simulink model "AutonomousTest1"  (R2021b)
settings: Solver=FixedStepAuto  StartTime=0.0  StopTime=inf  RelTol=1e-3
libraries: vexarmcortexlib x26, simulink x8, vexcommonlib x1
settings Model: SimulationMode=external  NumberOfSteps=6  Creator=arago  LastModifiedBy=arago
settings DataIOCC: LimitDataPoints=on  SignalLoggingSaveFormat=ModelDataLogs  ReturnWorkspaceOutputs=off
settings OptimizationCC: ExpressionDepthLimit=2147483647  LifeSpan=Inf  MaxStackSize=64  EfficientTunableParamExpr=on
settings DebuggingCC: UnderspecifiedInitializationDetection=Classic  MergeDetectMultiDrivingBlocksExec=none  InheritedTsInSrcMsg=none  FcnCallInpInsideContextMsg=warning  UnconnectedInputMsg=none  UnconnectedOutputMsg=none  StateNameClashWarn=warning  SFUnexpectedBacktrackingDiag=warning  SFNoUnconditionalDefaultTransitionDiag=warning  SFExecutionAtInitializationDiag=none  SFMachineParentedDataDiag=warning  ArithmeticOperatorsInVariantConditions=warning
settings HardwareCC: ProdBitPerPointer=32  ProdBitPerSizeT=32  ProdBitPerPtrDiffT=32  ProdLargestAtomicInteger=Long  ProdLargestAtomicFloat=Double  ProdIntDivRoundTo=Undefined  ProdWordSize=32  ProdHWDeviceType=ARM Compatible->ARM Cortex
settings ModelReferenceCC: PropagateSignalLabelsOutOfModel=off
settings SFSimCC: MATLABDynamicMemAlloc=off  CustomCodeUndefinedFunction=UseInterfaceOnly
settings RTWCC: Description=Embedded Coder  SystemTargetFile=ert.tlc  HardwareBoard=ARM Cortex-based VEX Microcontroller  TemplateMakefile=ert_default_tmf  Toolchain=GNU Tools for VEX ARM Cortex
settings CodeAppCC: IgnoreCustomStorageClasses=off  CustomSymbolStrType=$N$R$M  StateflowObjectComments=on  InternalIdentifier=Classic
settings ERTTargetCC: CodeReplacementLibrary=GCC ARM Cortex-M3  MultiwordLength=2048  ConvertIfToSwitch=off  SuppressUnreachableDefaultCases=off

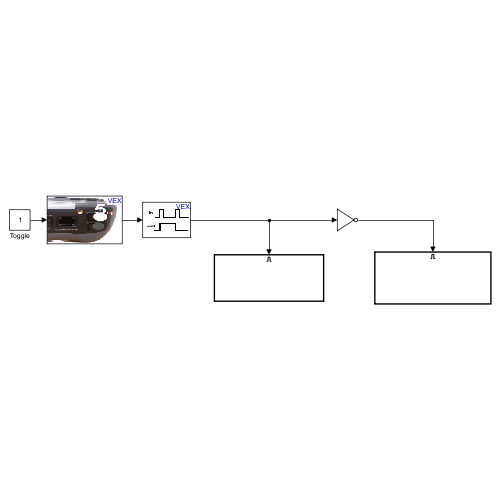
[thumbnail: Simulink's stored preview of the top-level diagram]
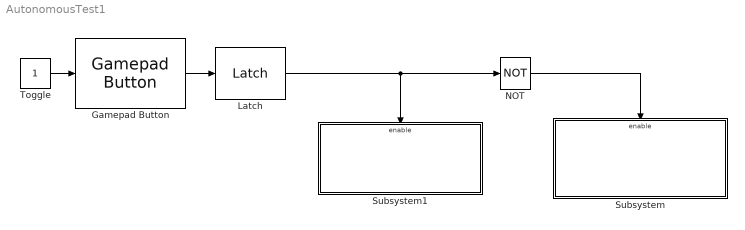
== system AutonomousTest1 ==
  Gamepad Button : vexarmcortexlib/Gamepad/Gamepad Button  joystick=1  chan=5  button56=Up  button78=Left  SimulationIn=on  SampleTime=0.02
      settings: SourceProductBaseCode=EC_VEX_MICRO
  Latch : vexcommonlib/Latch  output0=off  BlockPlatform=vexarmcortex
      settings: SourceProductBaseCode=EC_VEX_MICRO,VEXV5
  NOT : Logic  Operator=NOT  IconShape=distinctive  AllPortsSameDT=off  OutDataTypeStr=boolean
  Subsystem : Subsystem
  Subsystem1 : Subsystem
  Toggle : Constant
      settings: OpenFcn=|
      | if strcmp('0',get_param(gcb, 'Value'))                        set_param(gcb, 'Value', '1');
      | else
      |             set_param(gcb, 'Value', '0');
      | end
  wires:
  NOT/1 -> Subsystem/Enable
  Latch/1 -> Subsystem1/Enable, NOT/1
  Gamepad Button/1 -> Latch/1
  Toggle/1 -> Gamepad Button/1

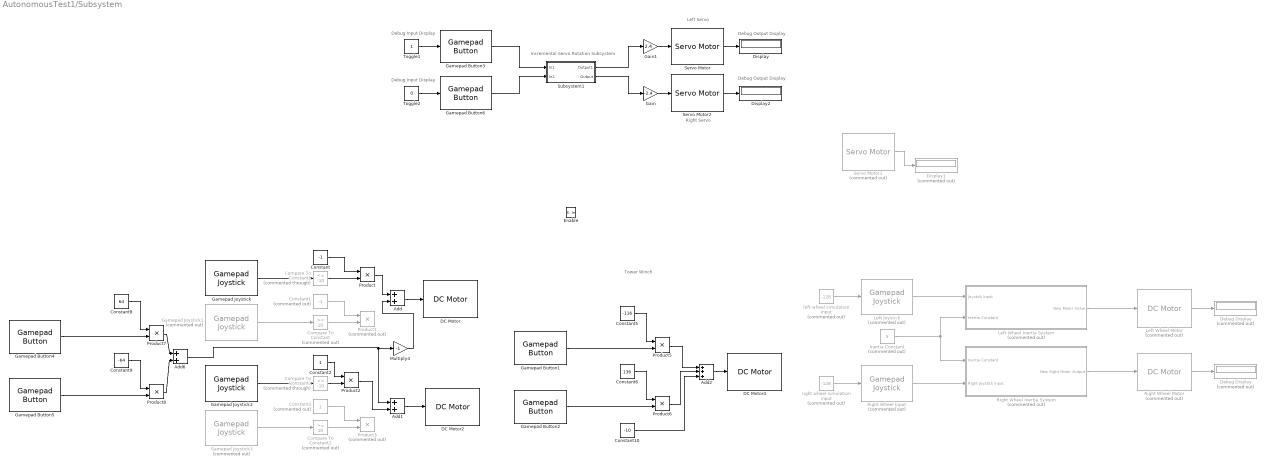
== system AutonomousTest1/Subsystem ==
  note: Incremental Servo Rotation Subsystem
  note: Left Servo
  note: Tower Winch
  note: Right Servo
  note: Debug Output Display
  note: Debug Output Display
  note: Debug Input Display
  note: Debug Input Display
  Enable : EnablePort
  " Debug Display" : Display  Commented=on
  Add : Sum
  Add1 : Sum
  Add2 : Sum  Inputs=+++
  Add6 : Sum
  Compare To Constant : simulink/Logic and Bit Operations/Compare To Constant  Commented=on  relop=>=  const=10  OutDataTypeStr=uint8
  Compare To Constant1 : simulink/Logic and Bit Operations/Compare To Constant  Commented=through  relop=<=  const=-10  OutDataTypeStr=uint8
  Compare To Constant2 : simulink/Logic and Bit Operations/Compare To Constant  Commented=on  relop=>=  const=10  OutDataTypeStr=uint8
  Compare To Constant3 : simulink/Logic and Bit Operations/Compare To Constant  Commented=through  relop=<=  const=-10  OutDataTypeStr=uint8
  Constant : Constant  Value=-1
  Constant1 : Constant  Commented=on  Value=-1
  Constant10 : Constant  Value=-10
  Constant2 : Constant
  Constant3 : Constant  Commented=on
  Constant5 : Constant  Value=-116
  Constant6 : Constant  Value=136
  Constant8 : Constant  Value=64
  Constant9 : Constant  Value=-64
  DC Motor : vexarmcortexlib/Actuators/DC Motor  motor=2  scaleFactor=1/13.5  SimulationOut=off
      settings: SourceProductBaseCode=EC_VEX_MICRO
  DC Motor2 : vexarmcortexlib/Actuators/DC Motor  motor=3  scaleFactor=1/13.5  SimulationOut=off
      settings: SourceProductBaseCode=EC_VEX_MICRO
  DC Motor4 : vexarmcortexlib/Actuators/DC Motor  motor=6  scaleFactor=1/13.5  SimulationOut=off
      settings: SourceProductBaseCode=EC_VEX_MICRO
  Debug Display : Display  Commented=on
  Display : Display
  Display1 : Display  Commented=on
  Display2 : Display
  Gain : Gain  Gain=-2.4
  Gain1 : Gain  Gain=2.4
  Gamepad Button1 : vexarmcortexlib/Gamepad/Gamepad Button  joystick=1  chan=8  button56=Up  button78=Up  SimulationIn=off  SampleTime=0.02
      settings: SourceProductBaseCode=EC_VEX_MICRO
  Gamepad Button2 : vexarmcortexlib/Gamepad/Gamepad Button  joystick=1  chan=8  button56=Up  button78=Down  SimulationIn=off  SampleTime=0.02
      settings: SourceProductBaseCode=EC_VEX_MICRO
  Gamepad Button3 : vexarmcortexlib/Gamepad/Gamepad Button  joystick=1  chan=6  button56=Up  button78=Down  SimulationIn=on  SampleTime=0.02
      settings: SourceProductBaseCode=EC_VEX_MICRO
  Gamepad Button4 : vexarmcortexlib/Gamepad/Gamepad Button  joystick=1  chan=7  button56=Up  button78=Up  SimulationIn=off  SampleTime=0.02
      settings: SourceProductBaseCode=EC_VEX_MICRO
  Gamepad Button5 : vexarmcortexlib/Gamepad/Gamepad Button  joystick=1  chan=7  button56=Up  button78=Down  SimulationIn=off  SampleTime=0.02
      settings: SourceProductBaseCode=EC_VEX_MICRO
  Gamepad Button6 : vexarmcortexlib/Gamepad/Gamepad Button  joystick=1  chan=6  button56=Down  button78=Down  SimulationIn=on  SampleTime=0.02
      settings: SourceProductBaseCode=EC_VEX_MICRO
  Gamepad Joystick : vexarmcortexlib/Gamepad/Gamepad Joystick  joystick=1  chan=2  SimulationIn=off  SampleTime=0.02
      settings: SourceProductBaseCode=EC_VEX_MICRO
  Gamepad Joystick1 : vexarmcortexlib/Gamepad/Gamepad Joystick  Commented=on  joystick=1  chan=2  SimulationIn=off  SampleTime=0.02
      settings: SourceProductBaseCode=EC_VEX_MICRO
  Gamepad Joystick2 : vexarmcortexlib/Gamepad/Gamepad Joystick  joystick=1  chan=3  SimulationIn=off  SampleTime=0.02
      settings: SourceProductBaseCode=EC_VEX_MICRO
  Gamepad Joystick3 : vexarmcortexlib/Gamepad/Gamepad Joystick  Commented=on  joystick=1  chan=3  SimulationIn=off  SampleTime=0.02
      settings: SourceProductBaseCode=EC_VEX_MICRO
  Inertia Constant : Constant  Commented=on  Value=5
  Left Joystick : vexarmcortexlib/Gamepad/Gamepad Joystick  Commented=on  joystick=1  chan=3  SimulationIn=on  SampleTime=0.02
      settings: SourceProductBaseCode=EC_VEX_MICRO
  Left Wheel Inertia System : Subsystem  Commented=on
  Left Wheel Motor : vexarmcortexlib/Actuators/DC Motor  Commented=on  motor=2  scaleFactor=1/13.5  SimulationOut=on
      settings: SourceProductBaseCode=EC_VEX_MICRO
  Multiply4 : Gain  Gain=-1
  Product{,2,5..8} (6 alike) : Product
  Product1 : Product  Commented=on
  Product3 : Product  Commented=on
  Right Wheel Inertia System : Subsystem  Commented=on
  Right Wheel Input : vexarmcortexlib/Gamepad/Gamepad Joystick  Commented=on  joystick=1  chan=2  SimulationIn=on  SampleTime=0.02
      settings: SourceProductBaseCode=EC_VEX_MICRO
  Right Wheel Motor : vexarmcortexlib/Actuators/DC Motor  Commented=on  motor=3  scaleFactor=1/13.5  SimulationOut=on
      settings: SourceProductBaseCode=EC_VEX_MICRO
  Servo Motor : vexarmcortexlib/Actuators/Servo Motor  motor=5  scaleFactor=60/127  SimulationOut=on
      settings: SourceProductBaseCode=EC_VEX_MICRO
  Servo Motor1 : vexarmcortexlib/Actuators/Servo Motor  Commented=on  motor=5  scaleFactor=60/127  SimulationOut=on
      settings: SourceProductBaseCode=EC_VEX_MICRO
  Servo Motor2 : vexarmcortexlib/Actuators/Servo Motor  motor=4  scaleFactor=60/127  SimulationOut=on
      settings: SourceProductBaseCode=EC_VEX_MICRO
  Subsystem1 : Subsystem
  Toggle1 : Constant
      settings: OpenFcn=|
      | if strcmp('0',get_param(gcb, 'Value'))                        set_param(gcb, 'Value', '1');
      | else
      |             set_param(gcb, 'Value', '0');
      | end
  Toggle2 : Constant  Value=0
      settings: OpenFcn=|
      | if strcmp('0',get_param(gcb, 'Value'))                        set_param(gcb, 'Value', '1');
      | else
      |             set_param(gcb, 'Value', '0');
      | end
  left wheel simulation input : Constant  Commented=on  Value=-128  SampleTime=0.02
  right wheel simulation input : Constant  Commented=on  Value=-128  SampleTime=0.02
  wires:
  Constant6/1 -> Product6/1
  Constant2/1 -> Product2/1
  Subsystem1/1(Output1) -> Gain1/1
  Constant10/1 -> Add2/3
  Gamepad Joystick1/1 -> Compare To Constant/1
  Product5/1 -> Add2/1
  Constant8/1 -> Product7/1
  Compare To Constant1/1 -> Product/2
  Gamepad Button3/1 -> Subsystem1/1(In1)
  Constant1/1 -> Product1/1
  Right Wheel Motor/1 -> Debug Display/1
  Constant5/1 -> Product5/1
  Servo Motor2/1 -> Display2/1
  Gamepad Joystick/1 -> Compare To Constant1/1
  right wheel simulation input/1 -> Right Wheel Input/1
  Product6/1 -> Add2/2
  left wheel simulation input/1 -> Left Joystick/1
  Servo Motor/1 -> Display/1
  Product2/1 -> Add1/2
  Gamepad Joystick3/1 -> Compare To Constant2/1
  Constant9/1 -> Product8/1
  Gamepad Button2/1 -> Product6/2
  Product/1 -> Add/1
  Compare To Constant/1 -> Product1/2
  Add2/1 -> DC Motor4/1
  Gamepad Button6/1 -> Subsystem1/2(In2)
  Compare To Constant2/1 -> Product3/2
  Left Wheel Motor/1 -> " Debug Display"/1
  Servo Motor1/1 -> Display1/1
  Constant/1 -> Product/1
  Add6/1 -> Multiply4/1, Add1/1
  Gamepad Button1/1 -> Product5/2
  Gamepad Joystick2/1 -> Compare To Constant3/1
  Compare To Constant3/1 -> Product2/2
  Product8/1 -> Add6/2
  Subsystem1/2(Output) -> Gain/1
  Product7/1 -> Add6/1
  Gain/1 -> Servo Motor2/1
  Constant3/1 -> Product3/1
  Inertia Constant/1 -> Right Wheel Inertia System/1(Inertia Constant), Left Wheel Inertia System/2(Inertia Constant)
  Gain1/1 -> Servo Motor/1
  Left Joystick/1 -> Left Wheel Inertia System/1(Joystick Input)
  Gamepad Button4/1 -> Product7/2
  Right Wheel Input/1 -> Right Wheel Inertia System/2(Right Joystick Input)
  Right Wheel Inertia System/1(New Right Motor Output) -> Right Wheel Motor/1
  Toggle2/1 -> Gamepad Button6/1
  Toggle1/1 -> Gamepad Button3/1
  Left Wheel Inertia System/1(New Motor Value) -> Left Wheel Motor/1
  Add1/1 -> DC Motor2/1
  Add/1 -> DC Motor/1
  Multiply4/1 -> Add/2
  Gamepad Button5/1 -> Product8/2

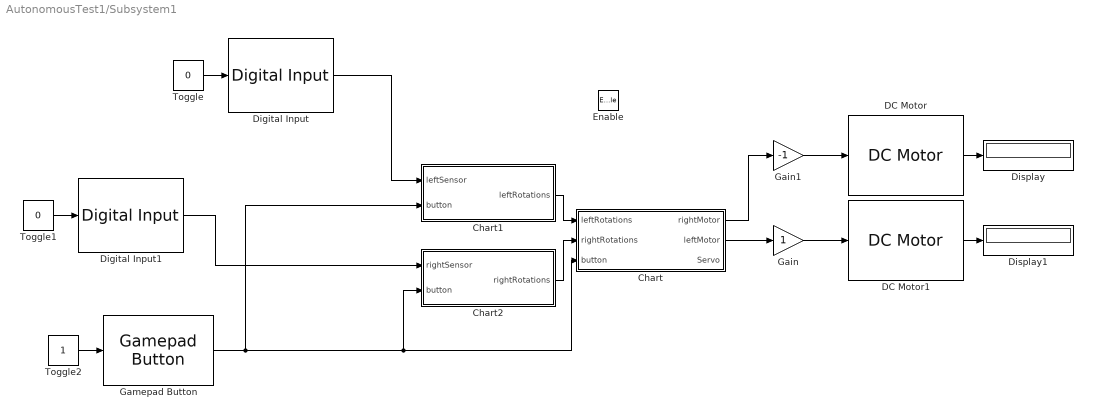
== system AutonomousTest1/Subsystem1 ==
  Enable : EnablePort
  Chart : Stateflow chart  TreatAsAtomicUnit=on
  Chart1 : Stateflow chart  TreatAsAtomicUnit=on
  Chart2 : Stateflow chart  TreatAsAtomicUnit=on
  DC Motor : vexarmcortexlib/Actuators/DC Motor  motor=2  scaleFactor=1/13.5  SimulationOut=on
      settings: SourceProductBaseCode=EC_VEX_MICRO
  DC Motor1 : vexarmcortexlib/Actuators/DC Motor  motor=3  scaleFactor=1/13.5  SimulationOut=on
      settings: SourceProductBaseCode=EC_VEX_MICRO
  Digital Input : vexarmcortexlib/Sensors/Digital Input  inChan=1  SimulationIn=on  SampleTime=.05
      settings: SourceProductBaseCode=EC_VEX_MICRO
  Digital Input1 : vexarmcortexlib/Sensors/Digital Input  inChan=2  SimulationIn=on  SampleTime=.05
      settings: SourceProductBaseCode=EC_VEX_MICRO
  Display : Display
  Display1 : Display
  Gain : Gain
  Gain1 : Gain  Gain=-1
  Gamepad Button : vexarmcortexlib/Gamepad/Gamepad Button  joystick=1  chan=5  button56=Up  button78=Left  SimulationIn=on  SampleTime=0.02
      settings: SourceProductBaseCode=EC_VEX_MICRO
  Toggle : Constant  Value=0
      settings: OpenFcn=|
      | if strcmp('0',get_param(gcb, 'Value'))                        set_param(gcb, 'Value', '1');
      | else
      |             set_param(gcb, 'Value', '0');
      | end
  Toggle1 : Constant  Value=0
      settings: OpenFcn=|
      | if strcmp('0',get_param(gcb, 'Value'))                        set_param(gcb, 'Value', '1');
      | else
      |             set_param(gcb, 'Value', '0');
      | end
  Toggle2 : Constant
      settings: OpenFcn=|
      | if strcmp('0',get_param(gcb, 'Value'))                        set_param(gcb, 'Value', '1');
      | else
      |             set_param(gcb, 'Value', '0');
      | end
  wires:
  Digital Input/1 -> Chart1/1(leftSensor)
  Chart1/1(leftRotations) -> Chart/1(leftRotations)
  Digital Input1/1 -> Chart2/1(rightSensor)
  Chart2/1(rightRotations) -> Chart/2(rightRotations)
  Gamepad Button/1 -> Chart2/2(button), Chart/3(button), Chart1/2(button)
  Toggle1/1 -> Digital Input1/1
  DC Motor/1 -> Display/1
  DC Motor1/1 -> Display1/1
  Chart/2(leftMotor) -> Gain/1
  Gain/1 -> DC Motor1/1
  Gain1/1 -> DC Motor/1
  Chart/1(rightMotor) -> Gain1/1
  Toggle2/1 -> Gamepad Button/1
  Toggle/1 -> Digital Input/1

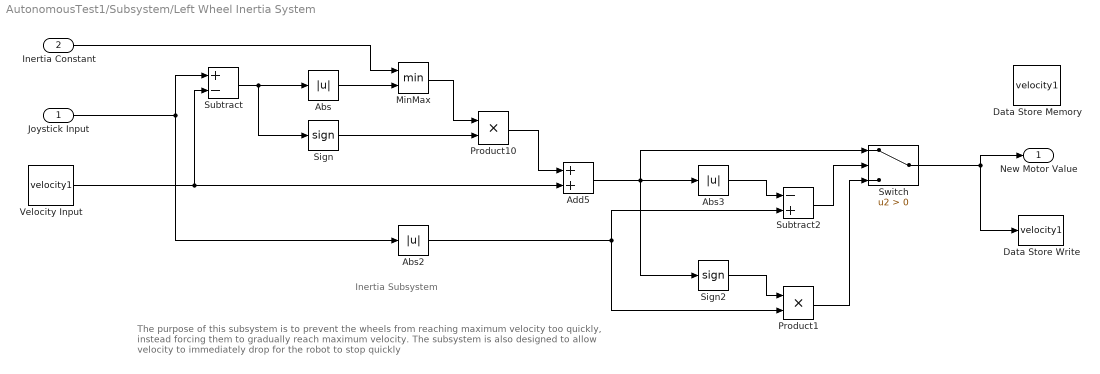
== system AutonomousTest1/Subsystem/Left Wheel Inertia System ==
  note: The purpose of this subsystem is to prevent the wheels from reaching maximum velocity too quickly, instead forcing them to gradually reach maximum velocity. The subsystem is also designed to allow velocity to immediately drop for the robot to stop quickly
  note: Inertia Subsystem
  Joystick Input : Inport
  Inertia Constant : Inport  Port=2
  Abs : Abs
  Abs2 : Abs
  Abs3 : Abs
  Add5 : Sum
  Data Store Memory : DataStoreMemory  DataStoreName=velocity1  ReadBeforeWriteMsg=warning  WriteAfterWriteMsg=warning  WriteAfterReadMsg=warning  ShowAdditionalParam=off
  Data Store Write : DataStoreWrite  DataStoreName=velocity1  SampleTime=0.02  IndexOptions=Index vector (dialog)  Indices=1  OutputSizes=1
  MinMax : MinMax  Inputs=2
  Product1 : Product  RndMeth=Zero
  Product10 : Product  RndMeth=Zero
  Sign : Signum
  Sign2 : Signum
  Subtract : Sum  Inputs=+-
  Subtract2 : Sum  Inputs=-+
  Switch : Switch  Criteria=u2 > Threshold
  Velocity Input : DataStoreRead  DataStoreName=velocity1  SampleTime=0.02  IndexOptions=Index vector (dialog)  Indices=1  OutputSizes=1
  New Motor Value : Outport
  wires:
  Joystick Input/1 -> Subtract/1, Abs2/1
  Subtract/1 -> Sign/1, Abs/1
  Add5/1 -> Sign2/1, Switch/1, Abs3/1
  Abs/1 -> MinMax/2
  Sign/1 -> Product10/2
  Velocity Input/1 -> Subtract/2, Add5/2
  Abs2/1 -> Subtract2/2, Product1/2
  Product10/1 -> Add5/1
  Sign2/1 -> Product1/1
  MinMax/1 -> Product10/1
  Inertia Constant/1 -> MinMax/1
  Switch/1 -> New Motor Value/1, Data Store Write/1
  Subtract2/1 -> Switch/2
  Abs3/1 -> Subtract2/1
  Product1/1 -> Switch/3

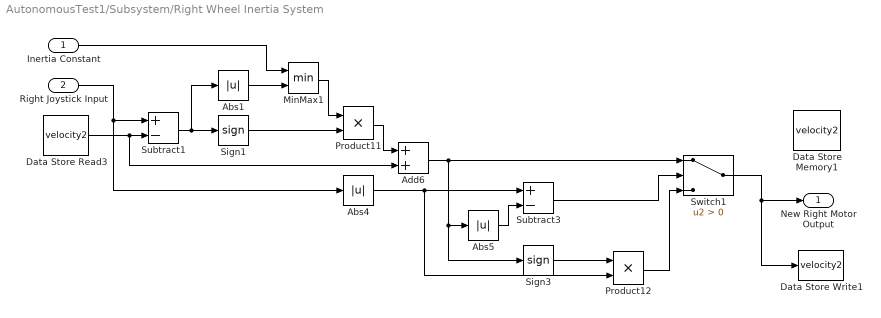
== system AutonomousTest1/Subsystem/Right Wheel Inertia System ==
  Inertia Constant : Inport
  Right Joystick Input : Inport  Port=2
  Abs1 : Abs
  Abs4 : Abs
  Abs5 : Abs
  Add6 : Sum
  Data Store Memory1 : DataStoreMemory  DataStoreName=velocity2  ReadBeforeWriteMsg=warning  WriteAfterWriteMsg=warning  WriteAfterReadMsg=warning  ShowAdditionalParam=off
  Data Store Read3 : DataStoreRead  DataStoreName=velocity2  SampleTime=0.02  IndexOptions=Index vector (dialog)  Indices=1  OutputSizes=1
  Data Store Write1 : DataStoreWrite  DataStoreName=velocity2  SampleTime=0.02  IndexOptions=Index vector (dialog)  Indices=1  OutputSizes=1
  MinMax1 : MinMax  Inputs=2
  Product11 : Product  RndMeth=Zero
  Product12 : Product  RndMeth=Zero
  Sign1 : Signum
  Sign3 : Signum
  Subtract1 : Sum  Inputs=+-
  Subtract3 : Sum  Inputs=+-
  Switch1 : Switch  Criteria=u2 > Threshold
  New Right Motor Output : Outport
  wires:
  MinMax1/1 -> Product11/1
  Abs5/1 -> Subtract3/2
  Product11/1 -> Add6/1
  Abs4/1 -> Product12/2, Subtract3/1
  Abs1/1 -> MinMax1/2
  Subtract3/1 -> Switch1/2
  Subtract1/1 -> Abs1/1, Sign1/1
  Sign1/1 -> Product11/2
  Sign3/1 -> Product12/1
  Data Store Read3/1 -> Subtract1/2, Add6/2
  Add6/1 -> Abs5/1, Sign3/1, Switch1/1
  Right Joystick Input/1 -> Abs4/1, Subtract1/1
  Inertia Constant/1 -> MinMax1/1
  Product12/1 -> Switch1/3
  Switch1/1 -> Data Store Write1/1, New Right Motor Output/1

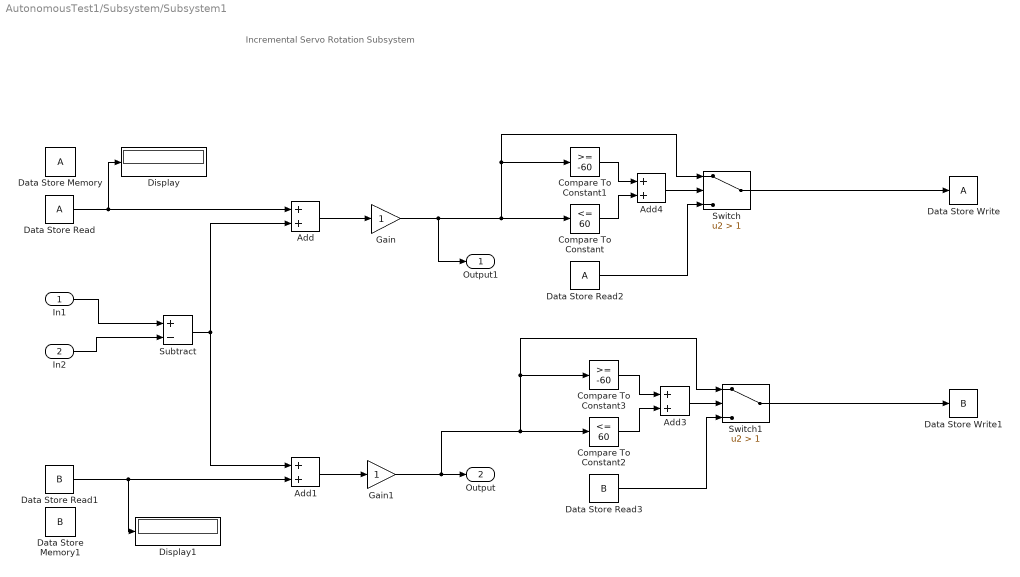
== system AutonomousTest1/Subsystem/Subsystem1 ==
  note: Incremental Servo Rotation Subsystem
  In1 : Inport
  In2 : Inport  Port=2
  Add{,1,3..4} (4 alike) : Sum
  Compare To Constant : simulink/Logic and Bit Operations/Compare To Constant  relop=<=  const=60  OutDataTypeStr=boolean
  Compare To Constant1 : simulink/Logic and Bit Operations/Compare To Constant  relop=>=  const=-60  OutDataTypeStr=boolean
  Compare To Constant2 : simulink/Logic and Bit Operations/Compare To Constant  relop=<=  const=60  OutDataTypeStr=boolean
  Compare To Constant3 : simulink/Logic and Bit Operations/Compare To Constant  relop=>=  const=-60  OutDataTypeStr=boolean
  Data Store Memory : DataStoreMemory  ReadBeforeWriteMsg=warning  WriteAfterWriteMsg=warning  WriteAfterReadMsg=warning  ShowAdditionalParam=off
  Data Store Memory1 : DataStoreMemory  DataStoreName=B  ReadBeforeWriteMsg=warning  WriteAfterWriteMsg=warning  WriteAfterReadMsg=warning  ShowAdditionalParam=off
  Data Store Read : DataStoreRead  IndexOptions=Index vector (dialog)  Indices=1  OutputSizes=1
  Data Store Read1 : DataStoreRead  DataStoreName=B  IndexOptions=Index vector (dialog)  Indices=1  OutputSizes=1
  Data Store Read2 : DataStoreRead  IndexOptions=Index vector (dialog)  Indices=1  OutputSizes=1
  Data Store Read3 : DataStoreRead  DataStoreName=B  IndexOptions=Index vector (dialog)  Indices=1  OutputSizes=1
  Data Store Write : DataStoreWrite  IndexOptions=Index vector (dialog)  Indices=1  OutputSizes=1
  Data Store Write1 : DataStoreWrite  DataStoreName=B  IndexOptions=Index vector (dialog)  Indices=1  OutputSizes=1
  Display : Display
  Display1 : Display
  Gain : Gain
  Gain1 : Gain
  Subtract : Sum  Inputs=+-
  Switch : Switch  Criteria=u2 > Threshold  Threshold=1
  Switch1 : Switch  Criteria=u2 > Threshold  Threshold=1
  Output1 : Outport
  Output : Outport  Port=2
  wires:
  In1/1 -> Subtract/1
  Add/1 -> Gain/1
  Add1/1 -> Gain1/1
  In2/1 -> Subtract/2
  Subtract/1 -> Add1/1, Add/2
  Gain/1 -> Compare To Constant1/1, Switch/1, Compare To Constant/1, Output1/1
  Switch/1 -> Data Store Write/1
  Switch1/1 -> Data Store Write1/1
  Data Store Read/1 -> Display/1, Add/1
  Data Store Read1/1 -> Display1/1, Add1/2
  Compare To Constant1/1 -> Add4/1
  Compare To Constant/1 -> Add4/2
  Add4/1 -> Switch/2
  Data Store Read2/1 -> Switch/3
  Compare To Constant2/1 -> Add3/2
  Data Store Read3/1 -> Switch1/3
  Add3/1 -> Switch1/2
  Compare To Constant3/1 -> Add3/1
  Gain1/1 -> Compare To Constant3/1, Switch1/1, Compare To Constant2/1, Output/1

== stateflow chart AutonomousTest1/Subsystem1/Chart ==
  state CloseClaw
    leftMotor = 0;
    rightMotor= 0;
    Servo = 0;
  state Straight
    leftMotor = 100;
    rightMotor = 100;
  state DriveForward
    leftMotor = 100;
    rightMotor = 100;
  state Right
    rightMotor = 100;
    leftMotor = 0;
  state Left
    rightMotor = 0;
    leftMotor = 100;
  state Stop
    leftMotor = 0;
    rightMotor = 0;
  state Turn
    leftMotor = -100;
    rightMotor = 100;
  CloseClaw -> Straight : [button == 1]
  DriveForward -> Straight [order 2] : [button == 1]
  (default) -> Straight
  Turn -> Straight [order 2] : [button == 1]
  Straight -> Right [order 3] : [leftRotations > (rightRotations)]
  DriveForward -> CloseClaw [order 1] : [rightRotations >= 19 || leftRotations >=16]
  Straight -> Left [order 2] : [rightRotations > (leftRotations)]
  Right -> Straight [order 3] : [rightRotations == leftRotations]
  Left -> Straight [order 2] : [rightRotations == leftRotations]
  Straight -> Stop [order 1] : [rightRotations >= 12 || leftRotations >= 12]
  Stop -> Straight [order 1] : [rightRotations<12 && leftRotations<12]
  Turn -> DriveForward [order 1] : after(0.5,sec)
  Right -> Left [order 1] : [rightRotations > (leftRotations)]
  Left -> Right [order 3] : [leftRotations > (rightRotations)]
  Right -> Stop [order 2] : [rightRotations >= 12 || leftRotations >= 12]
  Left -> Stop [order 1] : [rightRotations >= 12 || leftRotations >=12]
  Stop -> Turn [order 2] : after(2,sec)
  data: leftRotations input; rightRotations input; rightMotor output; leftMotor output; button input; Servo output

== stateflow chart AutonomousTest1/Subsystem1/Chart1 ==
  state OverBlack
    leftRotations = leftRotations + 1;
    leftFlag = 1;
  state Start
    leftRotations = 0;
  state Pause
    leftRotations;
  state OverWhite
    leftRotations = leftRotations + 1;
    leftFlag = 0;
  Start -> OverBlack [order 1] : [leftSensor == 0]
  OverBlack -> Pause
  Pause -> OverBlack [order 2] : [(leftSensor == 0) && (leftFlag == 0)]
  (default) -> Start
  Pause -> Start [order 1] : [button == 1]
  Start -> OverWhite [order 2] : [leftSensor == 1]
  Pause -> OverWhite [order 3] : [(leftSensor == 1) && (leftFlag == 1)]
  OverWhite -> Pause
  data: leftSensor input; leftFlag local; leftRotations output; button input

== stateflow chart AutonomousTest1/Subsystem1/Chart2 ==
  state OverBlack
    rightRotations = rightRotations + 1;
    rightFlag = 1;
  state Pause
    rightRotations;
  state Start
    rightRotations = 0;
  state OverWhite
    rightRotations = rightRotations + 1;
    rightFlag = 0;
  Pause -> OverBlack [order 2] : [(rightSensor == 0) && (rightFlag == 0)]
  Start -> OverBlack [order 1] : [rightSensor == 0]
  OverBlack -> Pause
  (default) -> Start
  Pause -> OverWhite [order 3] : [(rightSensor == 1) && (rightFlag == 1)]
  Pause -> Start [order 1] : [button == 1]
  OverWhite -> Pause
  Start -> OverWhite [order 2] : [rightSensor == 1]
  data: rightSensor input; rightRotations output; rightFlag local; button input
